simulink model "timeDelayedEKF_OOSM_2014a"  (R2015a)
settings: Solver=ode3  StartTime=0.0  StopTime=50  FixedStep=0.001  RelTol=1e-3
model workspace (MAT data in the model file):
  x_k = Simulink.Signal
  x_k.DataType = 'auto'
  x_k.Dimensions = [2 1]
  x_k.DimensionsMode = 'auto'
  x_k.Complexity = 'auto'
  x_k.SampleTime = -1
  x_k.SamplingMode = 'auto'
  x_k.InitialValue = '[0;0]'
  P_k = Simulink.Signal
  P_k.DataType = 'auto'
  P_k.Dimensions = [2 2]
  P_k.DimensionsMode = 'auto'
  P_k.Complexity = 'auto'
  P_k.SampleTime = -1
  P_k.SamplingMode = 'auto'
  P_k.InitialValue = '10*ones(2,2)'
  R = Simulink.Parameter
  R.Value = 0.001
  R.DataType = 'auto'
  t_delta = Simulink.Parameter
  t_delta.Value = 0.01
  t_delta.DataType = 'auto'
  x_d = Simulink.Signal
  x_d.DataType = 'auto'
  x_d.Dimensions = [2 1]
  x_d.DimensionsMode = 'auto'
  x_d.Complexity = 'auto'
  x_d.SampleTime = -1
  x_d.SamplingMode = 'auto'
  x_d.InitialValue = '[0;0]'
  P_d = Simulink.Signal
  P_d.DataType = 'auto'
  P_d.Dimensions = [2 2]
  P_d.DimensionsMode = 'auto'
  P_d.Complexity = 'auto'
  P_d.SampleTime = -1
  P_d.SamplingMode = 'auto'
  P_d.InitialValue = '10*eye(2,2)'
  U_n_d = Simulink.Signal
  U_n_d.DataType = 'auto'
  U_n_d.Dimensions = [2 2]
  U_n_d.DimensionsMode = 'auto'
  U_n_d.Complexity = 'auto'
  U_n_d.SampleTime = -1
  U_n_d.SamplingMode = 'auto'
  U_n_d.InitialValue = '10*eye(2,2)'
  FIFO_count = Simulink.Signal
  FIFO_count.DataType = 'auto'
  FIFO_count.Dimensions = 1
  FIFO_count.DimensionsMode = 'auto'
  FIFO_count.Complexity = 'auto'
  FIFO_count.SampleTime = -1
  FIFO_count.SamplingMode = 'auto'
  FIFO_count.InitialValue = '0'
undefined symbols (not defined in the file): des, gcbh
libraries: simulink x2
settings Model: PauseTimes=0  NumberOfSteps=10  CovSFcnEnable=off  Creator=Iseberg  LastModifiedBy=Ana
settings DebuggingCC: SolverPrmCheckMsg=warning

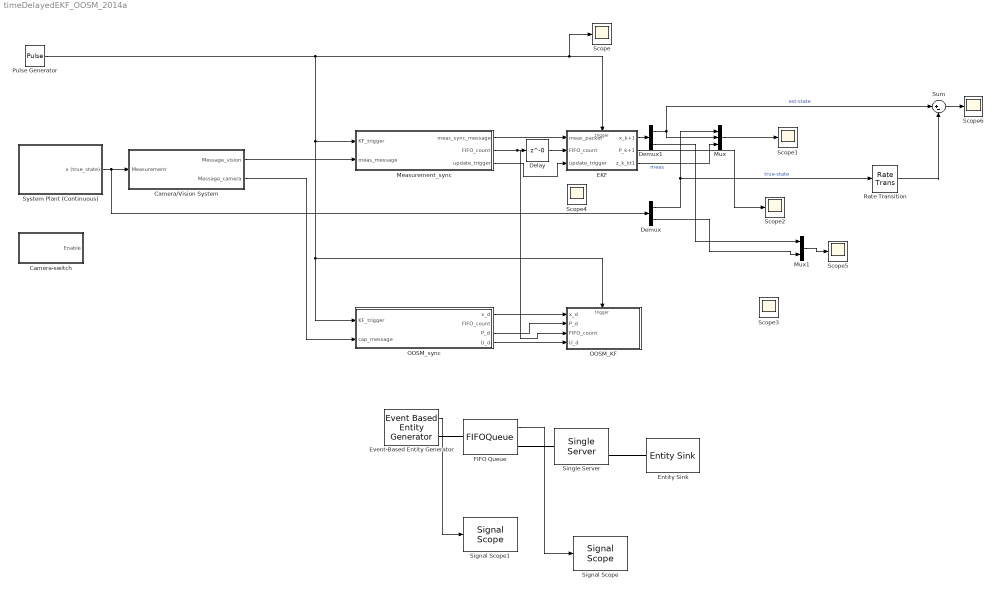
== system timeDelayedEKF_OOSM_2014a ==
  Camera-switch : Subsystem
  Camera/Vision System : Subsystem
  Delay : Delay  DelayLength=0  InitialCondition=0
  Demux : Demux  Outputs=2
  Demux1 : Demux  Outputs=2
  EKF : Subsystem  TreatAsAtomicUnit=on
  Entity Sink : EntitySink
  Event-Based Entity Generator : EventBasedEntityGenerator  GenerateEntitiesUpon=Function call from port fcn  StatNumberDeparted=on
  FIFO Queue : FIFOQueue  Capacity=1  StatNumberInBlock=on
      settings: OutputPortMap=o1
  Measurement_sync : Subsystem
  Mux : Mux  Inputs=3
  Mux1 : Mux  Inputs=2
  OOSM_KF : Subsystem  TreatAsAtomicUnit=on
  OOSM_sync : Subsystem
  Pulse Generator : DiscretePulseGenerator  Period=10  SampleTime=0.001
  Rate Transition : RateTransition
  Scope{,1..6} (7 alike) : Scope
      Scope settings: YMin=0  YMax=1
      Scope1 settings: ShowLegends=on  YMin=5  YMax=55  SaveName=ScopeData2
      Scope2 settings: YMin=0  YMax=21000  SaveName=ScopeData3
      Scope3 settings: YMin=0  YMax=1  SaveName=ScopeData4
      Scope4 settings: ShowLegends=on  YMin=-7.5e+263  YMax=3.25e+264  SaveName=ScopeData13
      Scope5 settings: ShowLegends=on  YMin=5  YMax=55  SaveName=ScopeData14
      Scope6 settings: YMin=0  YMax=1  SaveName=ScopeData15
  Signal Scope : SignalScope  LoadFcn=des.scope.CallbackSupport('seLoadFcn',gcbh)  StartFcn=des.scope.CallbackSupport('seStartFcn',gcbh)  StopFcn=des.scope.CallbackSupport('seStopFcn',gcbh)
      settings: CopyFcn=des.scope.CallbackSupport('seCopyFcn',gcbh)  DeleteFcn=des.scope.CallbackSupport('seDeleteFcn',gcbh)  PreSaveFcn=des.scope.CallbackSupport('sePreSaveFcn',gcbh)  NameChangeFcn=des.scope.CallbackSupport('seNameChangeFcn',gcbh)  OpenFcn=des.scope.CallbackSupport('seOpenFcn',gcbh)
  Signal Scope1 : SignalScope  LoadFcn=des.scope.CallbackSupport('seLoadFcn',gcbh)  StartFcn=des.scope.CallbackSupport('seStartFcn',gcbh)  StopFcn=des.scope.CallbackSupport('seStopFcn',gcbh)
      settings: CopyFcn=des.scope.CallbackSupport('seCopyFcn',gcbh)  DeleteFcn=des.scope.CallbackSupport('seDeleteFcn',gcbh)  PreSaveFcn=des.scope.CallbackSupport('sePreSaveFcn',gcbh)  NameChangeFcn=des.scope.CallbackSupport('seNameChangeFcn',gcbh)  OpenFcn=des.scope.CallbackSupport('seOpenFcn',gcbh)
  Single Server : SingleServer  StatNumberInBlock=on
      settings: OutputPortMap=o1
  Sum : Sum  Inputs=|+-
  System Plant (Continuous) : Subsystem
  wires:
  System Plant (Continuous)/1(x (true_state)) -> Demux/1, Camera/Vision System/1(Measurement)
  FIFO Queue/1 -> Signal Scope/1
  Event-Based Entity Generator/1 -> Signal Scope1/1
  Pulse Generator/1 -> Scope/1, EKF/Trigger, Measurement_sync/1(KF_trigger), OOSM_KF/Trigger, OOSM_sync/1(KF_trigger)
  Camera/Vision System/1("Message_vision ") -> Measurement_sync/2(meas_message)
  Measurement_sync/1(meas_sync_message) -> EKF/1(meas_packet)
  EKF/2("P_k+1 ") -> Scope2/1
  Mux/1 -> Scope1/1
  EKF/3(z_k_kt1) -> Mux/3  "meas"
  Camera/Vision System/2("Message_camera ") -> OOSM_sync/2(cap_message)
  OOSM_sync/1(x_d) -> OOSM_KF/1(x_d)
  OOSM_sync/3(P_d) -> OOSM_KF/2(P_d)
  Measurement_sync/2(FIFO_count) -> OOSM_KF/3(FIFO_count), Delay/1
  OOSM_sync/4(U_d) -> OOSM_KF/4(U_d)
  Demux/1 -> Rate Transition/1, Mux/1  "true-state"
  EKF/1(x_k+1) -> Demux1/1
  Demux1/1 -> Sum/1, Mux/2  "est-state"
  Delay/1 -> EKF/2(FIFO_count)
  Measurement_sync/3("update_trigger ") -> EKF/3("update_trigger ")
  Demux/2 -> Mux1/2
  Demux1/2 -> Mux1/1
  Mux1/1 -> Scope5/1
  Sum/1 -> Scope6/1
  Rate Transition/1 -> Sum/2
  connections:
  FIFO Queue/LConn1 -- Event-Based Entity Generator/RConn1
  Single Server/LConn1 -- FIFO Queue/RConn1
  Single Server/RConn1 -- Entity Sink/LConn1

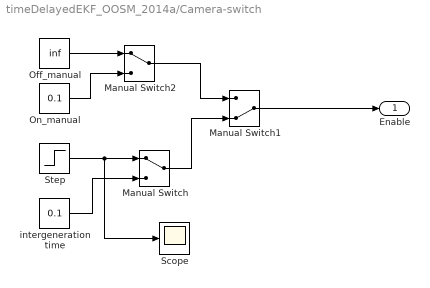
== system timeDelayedEKF_OOSM_2014a/Camera-switch ==
  Manual Switch : ManualSwitch
  Manual Switch1 : ManualSwitch  CurrentSetting=0
  Manual Switch2 : ManualSwitch
  Off_manual : Constant  Value=inf
  On_manual : Constant  Value=0.1
  Scope : Scope
      settings: SaveName=ScopeData6
  Step : Step  Time=abs(0.1*randn(1))  After=0.1  SampleTime=0
  intergeneration time : Constant  Value=0.1
  Enable : Outport
  wires:
  intergeneration time/1 -> Manual Switch/2
  Manual Switch2/1 -> Manual Switch1/1
  Off_manual/1 -> Manual Switch2/1
  Manual Switch1/1 -> Enable/1
  Step/1 -> Scope/1, Manual Switch/1
  Manual Switch/1 -> Manual Switch1/2
  On_manual/1 -> Manual Switch2/2

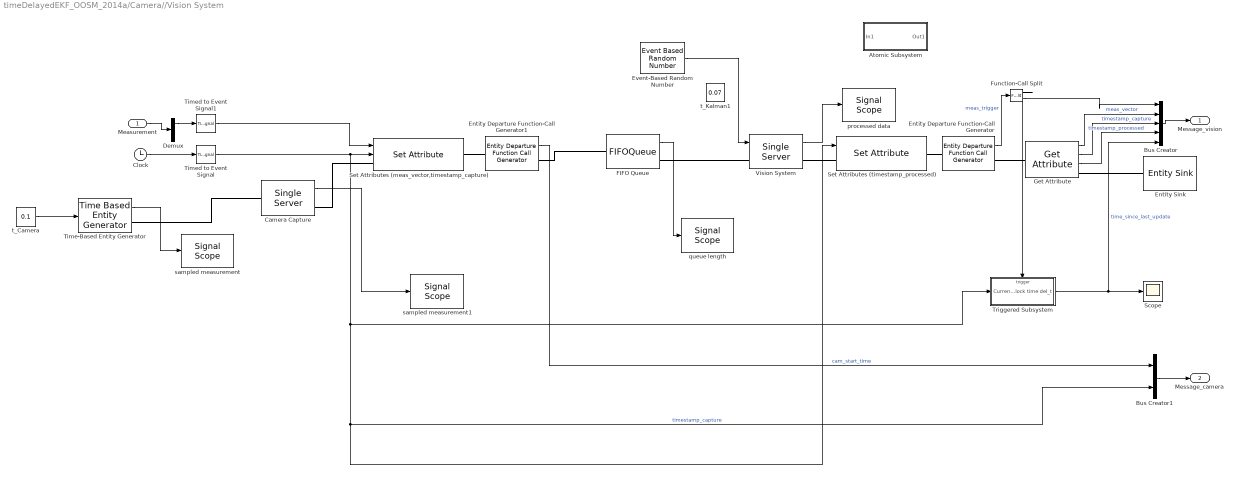
== system timeDelayedEKF_OOSM_2014a/Camera//Vision System ==
  Measurement : Inport
  Atomic Subsystem : Subsystem
  Bus Creator : BusCreator  Inputs=5
  Bus Creator1 : BusCreator  Inputs=2
  Camera Capture : SingleServer  ServiceTime=abs(0.01*randn(1))  StatNumberDeparted=on
  Clock : Clock
      settings: Decimation=2
  Demux : Demux  Outputs=2
  Entity Departure Function-Call Generator : EntityDepartureFunctionCallGenerator
  Entity Departure Function-Call Generator1 : EntityDepartureFunctionCallGenerator  TimingFunctionCallF1=Before entity departure
  Entity Sink : EntitySink
  Event-Based Random Number : EventBasedRandomNumber  Distribution=Uniform  minUnif=0.05  maxUnif=0.08
  FIFO Queue : FIFOQueue  Capacity=1  StatNumberInBlock=on
      settings: OutputPortMap=o1
  Function-Call Split : FunctionCallSplit
  Get Attribute : GetAttribute  AttributeName=meas_vector|timestamp_capture|timestamp_processed  AttributeMissing=Error|Error|Error  AttributeDefaultValue=1|1|1  AttributeTreatAsVector=1|1|1  AttributeSendTiming=After entity departure|After entity departure|After entity departure  EvaluatedDefaultAttributeValue={ [];[];[]}
      settings: OutputPortMap=o1,o2,o3
  Scope : Scope
  Set Attributes (meas_vector,timestamp_capture) : SetAttribute  AttributeName=meas_vector|timestamp_capture  AttributeFrom=Signal port|Signal port  AttributeValue=1|1  AttributeTreatAsVector=1|1  EvaluatedAttributeValue={ [];[]}
      settings: InputPortMap=u0,u1
  Set Attributes (timestamp_processed) : SetAttribute  AttributeName=timestamp_processed  AttributeFrom=Signal port  EvaluatedAttributeValue={ []}
  Time-Based Entity Generator : TimeBasedEntityGenerator  GenerateEntitiesUpon=Intergeneration time from port t  StatNumberDeparted=on
  Timed to Event Signal : TimedToEventSignal
  Timed to Event Signal1 : TimedToEventSignal
  Triggered Subsystem : Subsystem  TreatAsAtomicUnit=on
  "Vision System " : SingleServer  ServiceTimeFrom=Signal port t  StatNumberDeparted=on
  processed data : SignalScope  LoadFcn=des.scope.CallbackSupport('seLoadFcn',gcbh)  StartFcn=des.scope.CallbackSupport('seStartFcn',gcbh)  StopFcn=des.scope.CallbackSupport('seStopFcn',gcbh)
      settings: CopyFcn=des.scope.CallbackSupport('seCopyFcn',gcbh)  DeleteFcn=des.scope.CallbackSupport('seDeleteFcn',gcbh)  PreSaveFcn=des.scope.CallbackSupport('sePreSaveFcn',gcbh)  NameChangeFcn=des.scope.CallbackSupport('seNameChangeFcn',gcbh)  OpenFcn=des.scope.CallbackSupport('seOpenFcn',gcbh)
  queue length : SignalScope  LoadFcn=des.scope.CallbackSupport('seLoadFcn',gcbh)  StartFcn=des.scope.CallbackSupport('seStartFcn',gcbh)  StopFcn=des.scope.CallbackSupport('seStopFcn',gcbh)
      settings: CopyFcn=des.scope.CallbackSupport('seCopyFcn',gcbh)  DeleteFcn=des.scope.CallbackSupport('seDeleteFcn',gcbh)  PreSaveFcn=des.scope.CallbackSupport('sePreSaveFcn',gcbh)  NameChangeFcn=des.scope.CallbackSupport('seNameChangeFcn',gcbh)  OpenFcn=des.scope.CallbackSupport('seOpenFcn',gcbh)
  sampled measurement : SignalScope  LoadFcn=des.scope.CallbackSupport('seLoadFcn',gcbh)  StartFcn=des.scope.CallbackSupport('seStartFcn',gcbh)  StopFcn=des.scope.CallbackSupport('seStopFcn',gcbh)
      settings: CopyFcn=des.scope.CallbackSupport('seCopyFcn',gcbh)  DeleteFcn=des.scope.CallbackSupport('seDeleteFcn',gcbh)  PreSaveFcn=des.scope.CallbackSupport('sePreSaveFcn',gcbh)  NameChangeFcn=des.scope.CallbackSupport('seNameChangeFcn',gcbh)  OpenFcn=des.scope.CallbackSupport('seOpenFcn',gcbh)
  sampled measurement1 : SignalScope  LoadFcn=des.scope.CallbackSupport('seLoadFcn',gcbh)  StartFcn=des.scope.CallbackSupport('seStartFcn',gcbh)  StopFcn=des.scope.CallbackSupport('seStopFcn',gcbh)
      settings: CopyFcn=des.scope.CallbackSupport('seCopyFcn',gcbh)  DeleteFcn=des.scope.CallbackSupport('seDeleteFcn',gcbh)  PreSaveFcn=des.scope.CallbackSupport('sePreSaveFcn',gcbh)  NameChangeFcn=des.scope.CallbackSupport('seNameChangeFcn',gcbh)  OpenFcn=des.scope.CallbackSupport('seOpenFcn',gcbh)
  t_Camera : Constant  Value=0.1
  t_Kalman1 : Constant  Value=0.07
  "Message_vision " : Outport
  "Message_camera " : Outport  Port=2
  wires:
  Bus Creator/1 -> "Message_vision "/1
  Timed to Event Signal1/1 -> Set Attributes (meas_vector,timestamp_capture)/1
  Timed to Event Signal/1 -> Triggered Subsystem/1(Current Clock time), Bus Creator1/2, Set Attributes (timestamp_processed)/1, Set Attributes (meas_vector,timestamp_capture)/2  "timestamp_capture"
  Get Attribute/3 -> Bus Creator/4  "timestamp_processed"
  Time-Based Entity Generator/1 -> sampled measurement/1
  FIFO Queue/1 -> queue length/1
  "Vision System "/1 -> processed data/1
  Entity Departure Function-Call Generator/1 -> Function-Call Split/1  "meas_trigger"
  Get Attribute/2 -> Bus Creator/3  "timestamp_capture"
  Get Attribute/1 -> Bus Creator/2  "meas_vector"
  Clock/1 -> Timed to Event Signal/1
  Triggered Subsystem/1(del_t) -> Bus Creator/5, Scope/1  "time_since_last_update"
  Bus Creator1/1 -> "Message_camera "/1
  Entity Departure Function-Call Generator1/1 -> Bus Creator1/1  "cam_start_time"
  t_Camera/1 -> Time-Based Entity Generator/1
  Camera Capture/1 -> sampled measurement1/1
  Function-Call Split/2 -> Bus Creator/1
  Function-Call Split/1 -> Triggered Subsystem/Trigger
  Measurement/1 -> Demux/1
  Demux/1 -> Timed to Event Signal1/1
  Event-Based Random Number/1 -> "Vision System "/1
  connections:
  Entity Departure Function-Call Generator/LConn1 -- Set Attributes (timestamp_processed)/RConn1
  Get Attribute/RConn1 -- Entity Sink/LConn1
  "Vision System "/RConn1 -- Set Attributes (timestamp_processed)/LConn1
  Get Attribute/LConn1 -- Entity Departure Function-Call Generator/RConn1
  Entity Departure Function-Call Generator1/RConn1 -- FIFO Queue/LConn1
  Set Attributes (meas_vector,timestamp_capture)/RConn1 -- Entity Departure Function-Call Generator1/LConn1
  FIFO Queue/RConn1 -- "Vision System "/LConn1
  Camera Capture/LConn1 -- Time-Based Entity Generator/RConn1
  Camera Capture/RConn1 -- Set Attributes (meas_vector,timestamp_capture)/LConn1

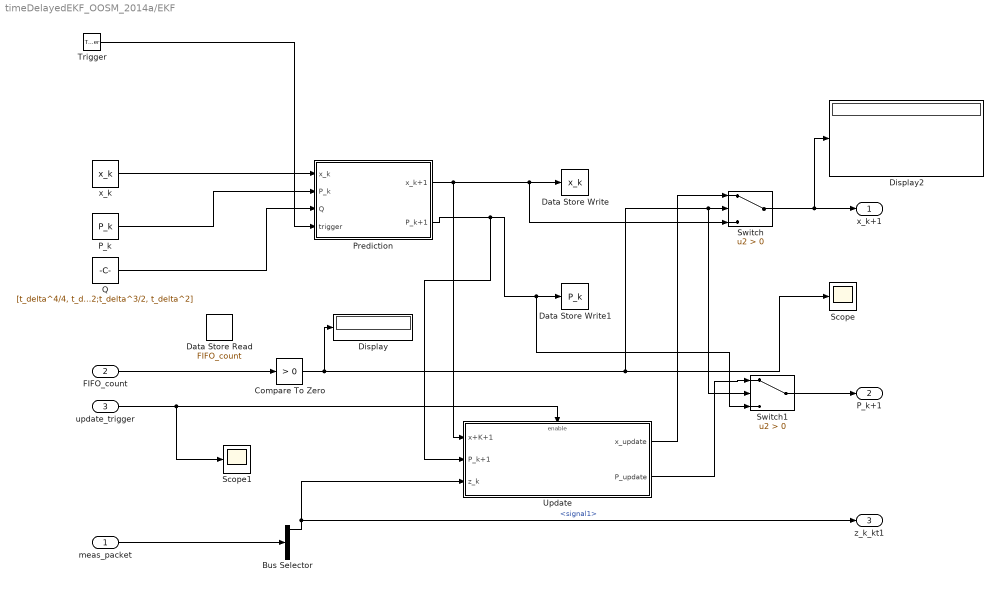
== system timeDelayedEKF_OOSM_2014a/EKF ==
  meas_packet : Inport
  FIFO_count : Inport  Port=2
  "update_trigger " : Inport  Port=3
  Trigger : TriggerPort  ShowOutputPort=on
  Bus Selector : BusSelector  OutputSignals=signal1,signal2,signal3,signal4
  Compare To Zero : simulink/Logic and Bit Operations/Compare To Zero  relop=>  OutDataTypeStr=uint8
  Data Store Read : DataStoreRead  DataStoreName=FIFO_count  DataStoreElements=FIFO_count
  Data Store Write : DataStoreWrite  DataStoreName=x_k  DataStoreElements=x_k
  Data Store Write1 : DataStoreWrite  DataStoreName=P_k  DataStoreElements=P_k
  Display : Display
  Display2 : Display
  P_k : DataStoreRead  DataStoreName=P_k  DataStoreElements=P_k
  Prediction : Subsystem
  Q : Constant  Value=[t_delta^4/4, t_delta^3/2;t_delta^3/2, t_delta^2]
  Scope : Scope
      settings: SaveName=ScopeData9
  Scope1 : Scope
      settings: SaveName=ScopeData12
  Switch : Switch  Criteria=u2 > Threshold
  Switch1 : Switch  Criteria=u2 > Threshold
  Update : Subsystem  TreatAsAtomicUnit=on
  x_k : DataStoreRead  DataStoreName=x_k  DataStoreElements=x_k
  x_k+1 : Outport
  "P_k+1 " : Outport  Port=2
  z_k_kt1 : Outport  Port=3
  wires:
  meas_packet/1 -> Bus Selector/1
  Prediction/2(P_k+1) -> Update/2(P_k+1), Switch1/3, Data Store Write1/1
  x_k/1 -> Prediction/1(x_k)
  P_k/1 -> Prediction/2(P_k)
  Q/1 -> Prediction/3(Q)
  Bus Selector/1 -> z_k_kt1/1, Update/3(z_k)  "<signal1>"
  Prediction/1(x_k+1) -> Switch/3, Data Store Write/1, Update/1(x+K+1)
  Update/1(x_update) -> Switch/1
  Switch/1 -> Display2/1, x_k+1/1
  Switch1/1 -> "P_k+1 "/1
  Trigger/1 -> Prediction/4(trigger)
  Update/2(P_update) -> Switch1/1
  FIFO_count/1 -> Compare To Zero/1
  Compare To Zero/1 -> Display/1, Switch1/2, Switch/2, Scope/1
  "update_trigger "/1 -> Scope1/1, Update/Enable

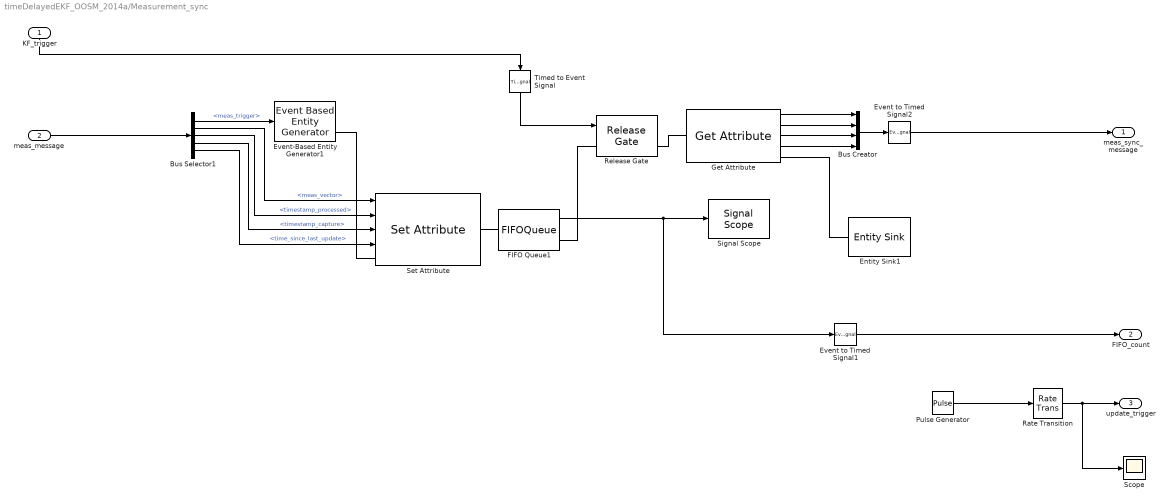
== system timeDelayedEKF_OOSM_2014a/Measurement_sync ==
  KF_trigger : Inport
  meas_message : Inport  Port=2
  Bus Creator : BusCreator
  Bus Selector1 : BusSelector  OutputSignals=meas_trigger,meas_vector,timestamp_processed,timestamp_capture,time_since_last_update
  Entity Sink1 : EntitySink
  Event to Timed Signal1 : EventToTimedSignal
  Event to Timed Signal2 : EventToTimedSignal
  Event-Based Entity Generator1 : EventBasedEntityGenerator  GenerateEntitiesUpon=Function call from port fcn  StatNumberDeparted=on
  FIFO Queue1 : FIFOQueue  Capacity=1  StatNumberInBlock=on
      settings: OutputPortMap=o1
  Get Attribute : GetAttribute  AttributeName=meas_vector|time_since_last_update|timestamp_capture|timestamp_processed  AttributeMissing=Error|Error|Error|Error  AttributeDefaultValue=1|1|1|1  AttributeTreatAsVector=1|1|1|1  AttributeSendTiming=After entity departure|After entity departure|After entity departure|After entity departure  EvaluatedDefaultAttributeValue={ [];[];[];[]}
      settings: OutputPortMap=o1,o2,o3,o4
  Pulse Generator : DiscretePulseGenerator  Period=100  PulseWidth=10  SampleTime=0.001
  Rate Transition : RateTransition
  Release Gate : ReleaseGate  StatNumberDeparted=on
  Scope : Scope
      settings: YMin=0  YMax=1  SaveName=ScopeData7
  Set Attribute : SetAttribute  AttributeName=meas_vector|timestamp_processed|timestamp_capture|time_since_last_update  AttributeFrom=Signal port|Signal port|Signal port|Signal port  AttributeValue=1|1|1|1  AttributeTreatAsVector=1|1|1|1  EvaluatedAttributeValue={ [];[];[];[]}
      settings: InputPortMap=u0,u1,u2,u3
  Signal Scope : SignalScope  LoadFcn=des.scope.CallbackSupport('seLoadFcn',gcbh)  StartFcn=des.scope.CallbackSupport('seStartFcn',gcbh)  StopFcn=des.scope.CallbackSupport('seStopFcn',gcbh)
      settings: CopyFcn=des.scope.CallbackSupport('seCopyFcn',gcbh)  DeleteFcn=des.scope.CallbackSupport('seDeleteFcn',gcbh)  PreSaveFcn=des.scope.CallbackSupport('sePreSaveFcn',gcbh)  NameChangeFcn=des.scope.CallbackSupport('seNameChangeFcn',gcbh)  OpenFcn=des.scope.CallbackSupport('seOpenFcn',gcbh)
  Timed to Event Signal : TimedToEventSignal
  meas_sync_message : Outport
  FIFO_count : Outport  Port=2
  "update_trigger " : Outport  Port=3
  wires:
  meas_message/1 -> Bus Selector1/1
  Get Attribute/4 -> Bus Creator/4
  Event to Timed Signal2/1 -> meas_sync_message/1
  Bus Selector1/1 -> Event-Based Entity Generator1/1  "<meas_trigger>"
  Get Attribute/3 -> Bus Creator/3
  Bus Selector1/2 -> Set Attribute/1  "<meas_vector>"
  Get Attribute/2 -> Bus Creator/2
  Timed to Event Signal/1 -> Release Gate/1
  Bus Creator/1 -> Event to Timed Signal2/1
  Get Attribute/1 -> Bus Creator/1
  KF_trigger/1 -> Timed to Event Signal/1
  Bus Selector1/5 -> Set Attribute/4  "<time_since_last_update>"
  Bus Selector1/3 -> Set Attribute/2  "<timestamp_processed>"
  Bus Selector1/4 -> Set Attribute/3  "<timestamp_capture>"
  FIFO Queue1/1 -> Event to Timed Signal1/1, Signal Scope/1
  Event to Timed Signal1/1 -> FIFO_count/1
  Pulse Generator/1 -> Rate Transition/1
  Rate Transition/1 -> Scope/1, "update_trigger "/1
  connections:
  Entity Sink1/LConn1 -- Get Attribute/RConn1
  FIFO Queue1/RConn1 -- Release Gate/LConn1
  Event-Based Entity Generator1/RConn1 -- Set Attribute/LConn1
  Get Attribute/LConn1 -- Release Gate/RConn1
  FIFO Queue1/LConn1 -- Set Attribute/RConn1

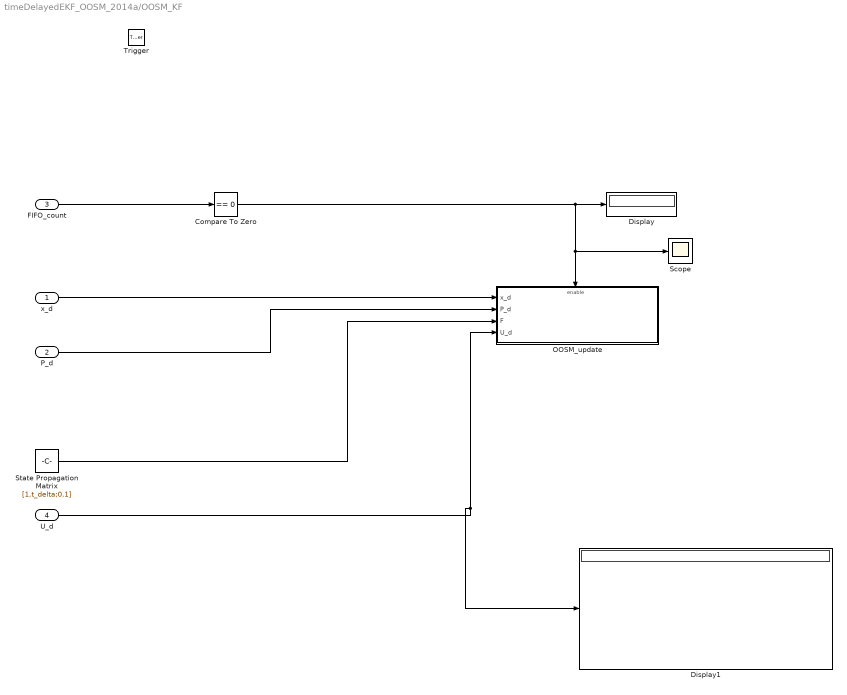
== system timeDelayedEKF_OOSM_2014a/OOSM_KF ==
  x_d : Inport
  P_d : Inport  Port=2
  FIFO_count : Inport  Port=3
  U_d : Inport  Port=4
  Trigger : TriggerPort
  Compare To Zero : simulink/Logic and Bit Operations/Compare To Zero  relop===  OutDataTypeStr=uint8
  Display : Display
  Display1 : Display
  OOSM_update : Subsystem
  Scope : Scope
      settings: SaveName=ScopeData8
  "State Propagation Matrix " : Constant  Value=[1,t_delta;0,1]
  wires:
  FIFO_count/1 -> Compare To Zero/1
  x_d/1 -> OOSM_update/1(x_d)
  P_d/1 -> OOSM_update/2(P_d)
  "State Propagation Matrix "/1 -> OOSM_update/3(F)
  Compare To Zero/1 -> OOSM_update/Enable, Scope/1, Display/1
  U_d/1 -> Display1/1, OOSM_update/4("U_d ")

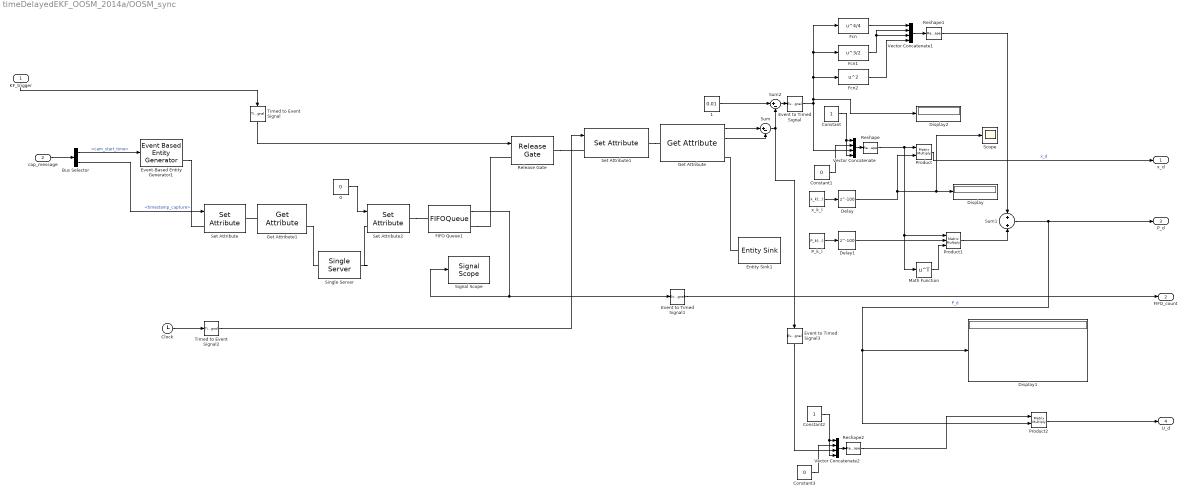
== system timeDelayedEKF_OOSM_2014a/OOSM_sync ==
  KF_trigger : Inport
  cap_message : Inport  Port=2
  0 : Constant  Value=0
  1 : Constant  Value=0.01
  Bus Selector : BusSelector  OutputSignals=cam_start_time,timestamp_capture
  Clock : Clock
  Constant : Constant
  Constant1 : Constant  Value=0
  Constant2 : Constant
  Constant3 : Constant  Value=0
  Delay : Delay  DelayLength=100  InitialCondition=0  SampleTime=0.001
  Delay1 : Delay  DelayLength=100  InitialCondition=10  SampleTime=0.001
  Display : Display
  Display1 : Display
  Display2 : Display
  Entity Sink1 : EntitySink
  Event to Timed Signal : EventToTimedSignal
  Event to Timed Signal1 : EventToTimedSignal
  Event to Timed Signal3 : EventToTimedSignal
  Event-Based Entity Generator1 : EventBasedEntityGenerator  GenerateEntitiesUpon=Function call from port fcn  StatNumberDeparted=on
  FIFO Queue1 : FIFOQueue  Capacity=5  StatNumberInBlock=on
      settings: OutputPortMap=o1
  Fcn : Fcn  Expr=u^4/4
  Fcn1 : Fcn  Expr=u^3/2
  Fcn2 : Fcn  Expr=u^2
  Get Attribute : GetAttribute  AttributeName=timestamp_KFTrigger|timestamp_capture|t_delta_oosm  AttributeMissing=Error|Error|Error  AttributeDefaultValue=1|1|1  AttributeTreatAsVector=1|1|1  AttributeSendTiming=After entity departure|After entity departure|After entity departure  EvaluatedDefaultAttributeValue={ [];[];[]}
      settings: OutputPortMap=o1,o2,o3
  Get Attribute1 : GetAttribute  AttributeName=timestamp_capture  EvaluatedDefaultAttributeValue={ []}
      settings: OutputPortMap=o1
  Math Function : Math  Operator=transpose  SaturateOnIntegerOverflow=on
  P_k_l : DataStoreRead  DataStoreName=P_k  DataStoreElements=P_k(:,:)
  Product : Product  Multiplication=Matrix(*)
  Product1 : Product  Inputs=3  Multiplication=Matrix(*)
  Product2 : Product  Multiplication=Matrix(*)
  Release Gate : ReleaseGate
  Reshape : Reshape  OutputDimensionality=Customize  OutputDimensions=[2,2]
  Reshape1 : Reshape  OutputDimensionality=Customize  OutputDimensions=[2,2]
  Reshape2 : Reshape  OutputDimensionality=Customize  OutputDimensions=[2,2]
  Scope : Scope
      settings: SaveName=ScopeData10
  Set Attribute : SetAttribute  AttributeName=timestamp_capture  AttributeFrom=Signal port  EvaluatedAttributeValue={ []}
  Set Attribute1 : SetAttribute  AttributeName=timestamp_KFTrigger  AttributeFrom=Signal port  EvaluatedAttributeValue={ []}
  Set Attribute2 : SetAttribute  AttributeName=t_delta_oosm  AttributeFrom=Signal port  EvaluatedAttributeValue={ []}
  Signal Scope : SignalScope  LoadFcn=des.scope.CallbackSupport('seLoadFcn',gcbh)  StartFcn=des.scope.CallbackSupport('seStartFcn',gcbh)  StopFcn=des.scope.CallbackSupport('seStopFcn',gcbh)
      settings: CopyFcn=des.scope.CallbackSupport('seCopyFcn',gcbh)  DeleteFcn=des.scope.CallbackSupport('seDeleteFcn',gcbh)  PreSaveFcn=des.scope.CallbackSupport('sePreSaveFcn',gcbh)  NameChangeFcn=des.scope.CallbackSupport('seNameChangeFcn',gcbh)  OpenFcn=des.scope.CallbackSupport('seOpenFcn',gcbh)
  Single Server : SingleServer  ServiceTime=0
  Sum : Sum  Inputs=|+-
  Sum1 : Sum
  Sum2 : Sum  Inputs=|+-
  Timed to Event Signal : TimedToEventSignal
  Timed to Event Signal2 : TimedToEventSignal
  Vector Concatenate : Concatenate  NumInputs=4
  Vector Concatenate1 : Concatenate  NumInputs=4
  Vector Concatenate2 : Concatenate  NumInputs=4
  x_k_l : DataStoreRead  DataStoreName=x_k  DataStoreElements=x_k(:,:)
  x_d : Outport
  FIFO_count : Outport  Port=2
  P_d : Outport  Port=3
  U_d : Outport  Port=4
  wires:
  Event to Timed Signal1/1 -> FIFO_count/1
  FIFO Queue1/1 -> Event to Timed Signal1/1, Signal Scope/1
  KF_trigger/1 -> Timed to Event Signal/1
  Timed to Event Signal/1 -> Release Gate/1
  cap_message/1 -> Bus Selector/1
  Bus Selector/1 -> Event-Based Entity Generator1/1  "<cam_start_time>"
  Bus Selector/2 -> Set Attribute/1  "<timestamp_capture>"
  Clock/1 -> Timed to Event Signal2/1
  Timed to Event Signal2/1 -> Set Attribute1/1
  Get Attribute/1 -> Sum/1
  Get Attribute/2 -> Sum/2
  Constant/1 -> Vector Concatenate/4, Vector Concatenate/1
  Constant1/1 -> Vector Concatenate/2
  Vector Concatenate/1 -> Reshape/1
  Math Function/1 -> Product1/3
  Fcn/1 -> Vector Concatenate1/1
  Fcn1/1 -> Vector Concatenate1/3, Vector Concatenate1/2
  Fcn2/1 -> Vector Concatenate1/4
  Vector Concatenate1/1 -> Reshape1/1
  Product1/1 -> Sum1/2
  0/1 -> Set Attribute2/1
  1/1 -> Sum2/1
  Event to Timed Signal/1 -> Display2/1, Fcn2/1, Fcn1/1, Fcn/1, Vector Concatenate/3
  Product/1 -> x_d/1  "x_d"
  Sum2/1 -> Event to Timed Signal/1
  Reshape1/1 -> Sum1/1
  Sum1/1 -> Product2/2, Display1/1, P_d/1  "P_d"
  Delay/1 -> Product/2, Scope/1, Display/1
  Delay1/1 -> Product1/2
  P_k_l/1 -> Delay1/1
  x_k_l/1 -> Delay/1
  Reshape/1 -> Product1/1, Math Function/1, Product/1
  Product2/1 -> U_d/1
  Constant2/1 -> Vector Concatenate2/4, Vector Concatenate2/1
  Constant3/1 -> Vector Concatenate2/2
  Vector Concatenate2/1 -> Reshape2/1
  Sum/1 -> Sum2/2, Event to Timed Signal3/1
  Reshape2/1 -> Product2/1
  Event to Timed Signal3/1 -> Vector Concatenate2/3
  connections:
  Event-Based Entity Generator1/RConn1 -- Set Attribute/LConn1
  FIFO Queue1/RConn1 -- Release Gate/LConn1
  Entity Sink1/LConn1 -- Get Attribute/RConn1
  Release Gate/RConn1 -- Set Attribute1/LConn1
  Set Attribute1/RConn1 -- Get Attribute/LConn1
  Get Attribute1/LConn1 -- Set Attribute/RConn1
  Set Attribute2/RConn1 -- FIFO Queue1/LConn1
  Get Attribute1/RConn1 -- Single Server/LConn1
  Single Server/RConn1 -- Set Attribute2/LConn1

== system timeDelayedEKF_OOSM_2014a/System Plant (Continuous) ==
  Integrator : Integrator  InitialConditionSource=external
  Product1 : Product  Multiplication=Matrix(*)
  State Matrix 1 : Constant  Value=[5;1]
  State Matrix 2 : Constant  Value=[0,1;0,0]
  x (true_state) : Outport
  wires:
  State Matrix 1/1 -> Integrator/2
  State Matrix 2/1 -> Product1/1
  Integrator/1 -> x (true_state)/1, Product1/2
  Product1/1 -> Integrator/1

== system timeDelayedEKF_OOSM_2014a/Camera//Vision System/Atomic Subsystem ==
  In1 : Inport
  Constant : Constant  Value=100
  Gain : Gain  Gain=100
  Product : Product
  Rounding Function : Rounding
  Scope : Scope
      settings: SaveName=ScopeData5
  Out1 : Outport
  wires:
  In1/1 -> Gain/1
  Gain/1 -> Rounding Function/1
  Constant/1 -> Product/2
  Product/1 -> Scope/1, Out1/1
  Rounding Function/1 -> Product/1

== system timeDelayedEKF_OOSM_2014a/Camera//Vision System/Triggered Subsystem ==
  Current Clock time : Inport
  Trigger : TriggerPort  TriggerType=function-call
  Delay : Delay  DelayLength=1  InitialCondition=0
  Sum : Sum  Inputs=|+-
  del_t : Outport
  wires:
  Current Clock time/1 -> Sum/1, Delay/1
  Sum/1 -> del_t/1
  Delay/1 -> Sum/2

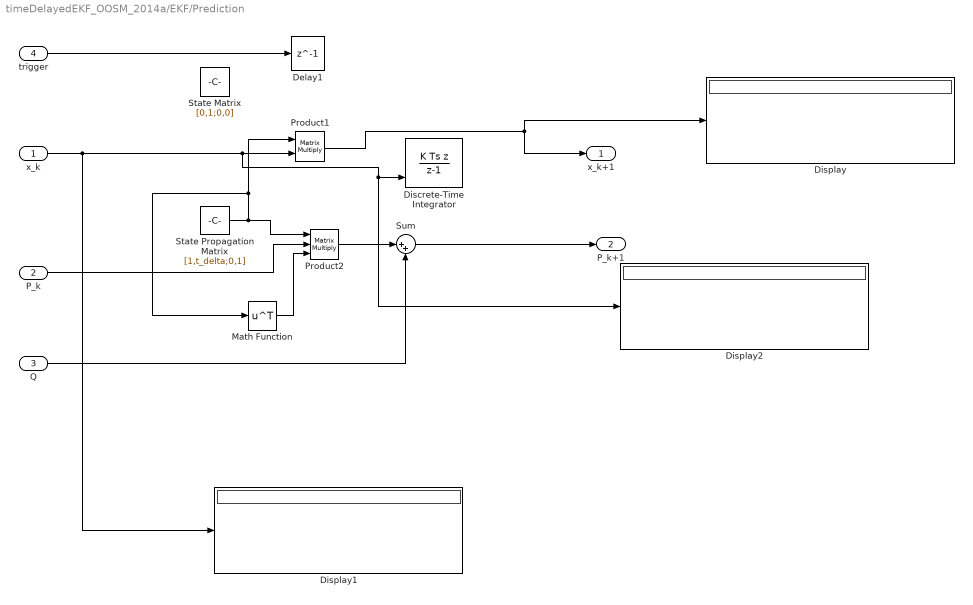
== system timeDelayedEKF_OOSM_2014a/EKF/Prediction ==
  x_k : Inport
  P_k : Inport  Port=2
  Q : Inport  Port=3
  trigger : Inport  Port=4
  Delay1 : Delay  DelayLength=1  InitialCondition=0
  Discrete-Time Integrator : DiscreteIntegrator  IntegratorMethod=Integration: Backward Euler  ExternalReset=rising  InitialConditionSource=external  InitialCondition=x_k  SampleTime=-1
  Display : Display
  Display1 : Display
  Display2 : Display
  Math Function : Math  Operator=transpose  SaturateOnIntegerOverflow=on
  Product1 : Product  Multiplication=Matrix(*)
  Product2 : Product  Inputs=3  Multiplication=Matrix(*)
  State Matrix : Constant  Value=[0,1;0,0]
  "State Propagation Matrix " : Constant  Value=[1,t_delta;0,1]
  Sum : Sum  Inputs=|++
  x_k+1 : Outport
  P_k+1 : Outport  Port=2
  wires:
  Product2/1 -> Sum/1
  Q/1 -> Sum/2
  P_k/1 -> Product2/2
  Sum/1 -> P_k+1/1
  "State Propagation Matrix "/1 -> Product1/1, Math Function/1, Product2/1
  Math Function/1 -> Product2/3
  trigger/1 -> Delay1/1
  x_k/1 -> Display1/1, Display2/1, Discrete-Time Integrator/3, Product1/2
  Product1/1 -> x_k+1/1, Display/1

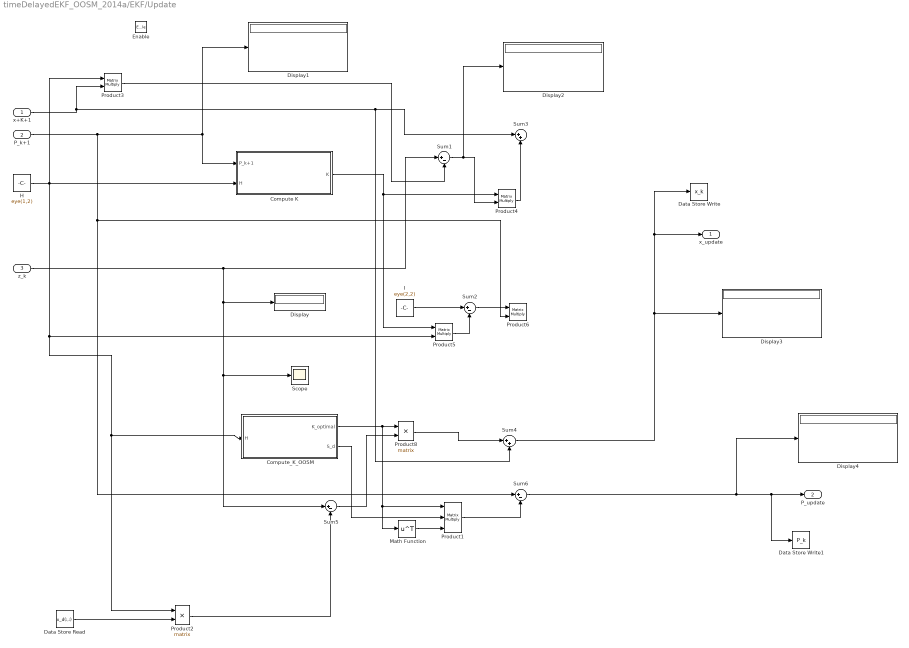
== system timeDelayedEKF_OOSM_2014a/EKF/Update ==
  x+K+1 : Inport
  P_k+1 : Inport  Port=2
  z_k : Inport  Port=3
  Enable : EnablePort
  Compute K : Subsystem
  Compute_K_OOSM : Subsystem
  Data Store Read : DataStoreRead  DataStoreName=x_d  DataStoreElements=x_d(:,:)
  Data Store Write : DataStoreWrite  DataStoreName=x_k
  Data Store Write1 : DataStoreWrite  DataStoreName=P_k
  Display{,1..4} (5 alike) : Display
  H : Constant  Value=eye(1,2)  VectorParams1D=off
  I : Constant  Value=eye(2,2)
  Math Function : Math  Operator=transpose  SaturateOnIntegerOverflow=on
  Product1 : Product  Inputs=3  Multiplication=Matrix(*)
  Product{2..6,8} (6 alike) : Product  Multiplication=Matrix(*)
  Scope : Scope
      settings: TimeRange=5  SaveName=ScopeData11
  Sum{1..2,5..6} (4 alike) : Sum  Inputs=|+-
  Sum3 : Sum  Inputs=|++
  Sum4 : Sum  Inputs=|++
  x_update : Outport
  P_update : Outport  Port=2
  wires:
  P_k+1/1 -> Sum6/1, Product6/2, Compute K/1(P_k+1), Display1/1
  H/1 -> Product2/1, Compute_K_OOSM/1(H), Product5/2, Compute K/2(H), Product3/1
  x+K+1/1 -> Sum4/2, Sum3/1, Product3/2
  z_k/1 -> Sum1/1, Display/1, Scope/1, Sum5/1
  Product3/1 -> Sum1/2
  Sum1/1 -> Display2/1, Product4/2
  Product4/1 -> Sum3/2
  I/1 -> Sum2/1
  Product5/1 -> Sum2/2
  Sum2/1 -> Product6/1
  Sum6/1 -> Display4/1, Data Store Write1/1, P_update/1
  Sum4/1 -> Data Store Write/1, x_update/1, Display3/1
  Compute K/1(K) -> Product5/1, Product4/1
  Data Store Read/1 -> Product2/2
  Product2/1 -> Sum5/2
  Compute_K_OOSM/1(K_optimal) -> Product1/1, Math Function/1, Product8/1
  Sum5/1 -> Product8/2
  Product8/1 -> Sum4/1
  Compute_K_OOSM/2(S_d) -> Product1/2
  Math Function/1 -> Product1/3
  Product1/1 -> Sum6/2

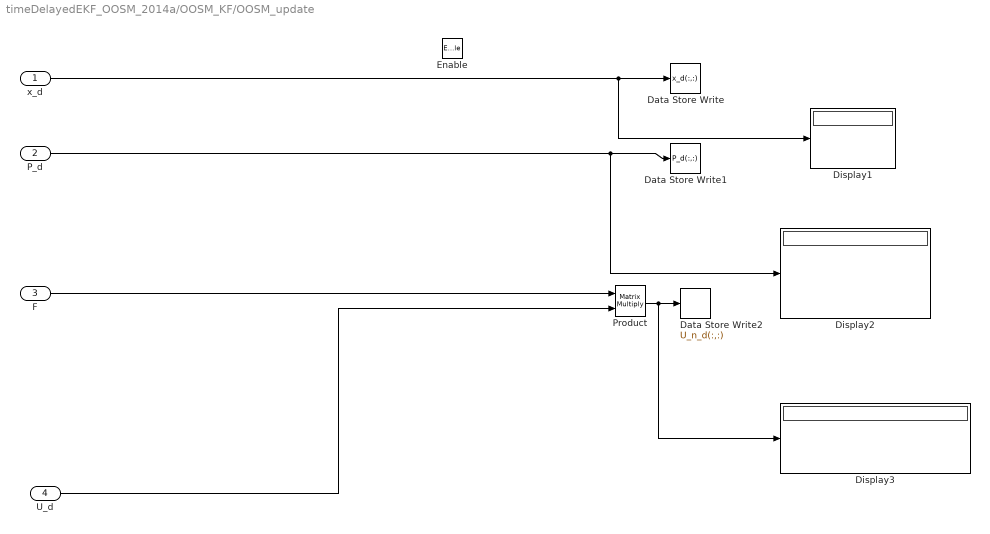
== system timeDelayedEKF_OOSM_2014a/OOSM_KF/OOSM_update ==
  x_d : Inport
  P_d : Inport  Port=2
  F : Inport  Port=3
  "U_d " : Inport  Port=4
  Enable : EnablePort
  Data Store Write : DataStoreWrite  DataStoreName=x_d  DataStoreElements=x_d(:,:)
  Data Store Write1 : DataStoreWrite  DataStoreName=P_d  DataStoreElements=P_d(:,:)
  Data Store Write2 : DataStoreWrite  DataStoreName=U_n_d  DataStoreElements=U_n_d(:,:)
  Display1 : Display
  Display2 : Display
  Display3 : Display
  Product : Product  Multiplication=Matrix(*)
  wires:
  F/1 -> Product/1
  x_d/1 -> Display1/1, Data Store Write/1
  Product/1 -> Display3/1, Data Store Write2/1
  P_d/1 -> Display2/1, Data Store Write1/1
  "U_d "/1 -> Product/2

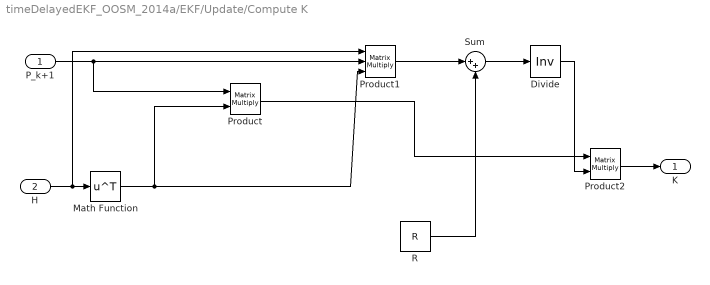
== system timeDelayedEKF_OOSM_2014a/EKF/Update/Compute K ==
  P_k+1 : Inport
  H : Inport  Port=2
  Divide : Product  Inputs=/  Multiplication=Matrix(*)
  Math Function : Math  Operator=transpose  SaturateOnIntegerOverflow=on
  Product : Product  Multiplication=Matrix(*)
  Product1 : Product  Inputs=3  Multiplication=Matrix(*)
  Product2 : Product  Multiplication=Matrix(*)
  R : Constant  Value=R
  Sum : Sum  Inputs=|++
  K : Outport
  wires:
  P_k+1/1 -> Product/1, Product1/2
  H/1 -> Product1/1, Math Function/1
  Sum/1 -> Divide/1
  Product1/1 -> Sum/1
  Divide/1 -> Product2/2
  Product2/1 -> K/1
  Product/1 -> Product2/1
  Math Function/1 -> Product/2, Product1/3
  R/1 -> Sum/2

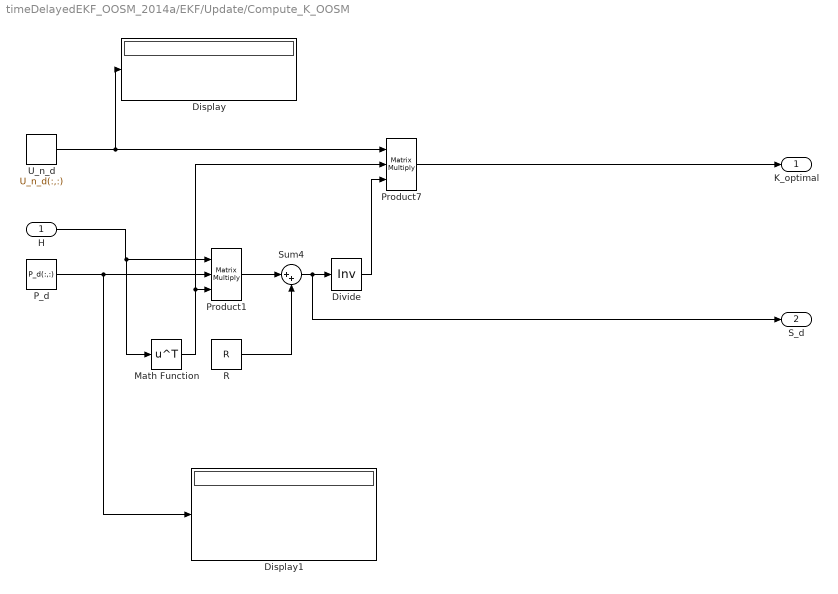
== system timeDelayedEKF_OOSM_2014a/EKF/Update/Compute_K_OOSM ==
  H : Inport
  Display : Display
  Display1 : Display
  Divide : Product  Inputs=/  Multiplication=Matrix(*)
  Math Function : Math  Operator=transpose  SaturateOnIntegerOverflow=on
  P_d : DataStoreRead  DataStoreName=P_d  DataStoreElements=P_d(:,:)
  Product1 : Product  Inputs=3  Multiplication=Matrix(*)
  Product7 : Product  Inputs=3  Multiplication=Matrix(*)
  R : Constant  Value=R
  Sum4 : Sum  Inputs=|++
  U_n_d : DataStoreRead  DataStoreName=U_n_d  DataStoreElements=U_n_d(:,:)
  K_optimal : Outport
  S_d : Outport  Port=2
  wires:
  Math Function/1 -> Product7/2, Product1/3
  R/1 -> Sum4/2
  U_n_d/1 -> Display/1, Product7/1
  P_d/1 -> Display1/1, Product1/2
  Product1/1 -> Sum4/1
  H/1 -> Math Function/1, Product1/1
  Product7/1 -> K_optimal/1
  Divide/1 -> Product7/3
  Sum4/1 -> S_d/1, Divide/1
